simulink model "Regressao6"  (R2012b)
settings: Solver=FixedStepDiscrete  SolverMode=SingleTasking  StartTime=0.0  StopTime=limSim  FixedStep=ts  RelTol=1e-3
libraries: xbsIndex_r4 x51, roblocks x1
settings Model: Creator=snata  LastModifiedBy=snata

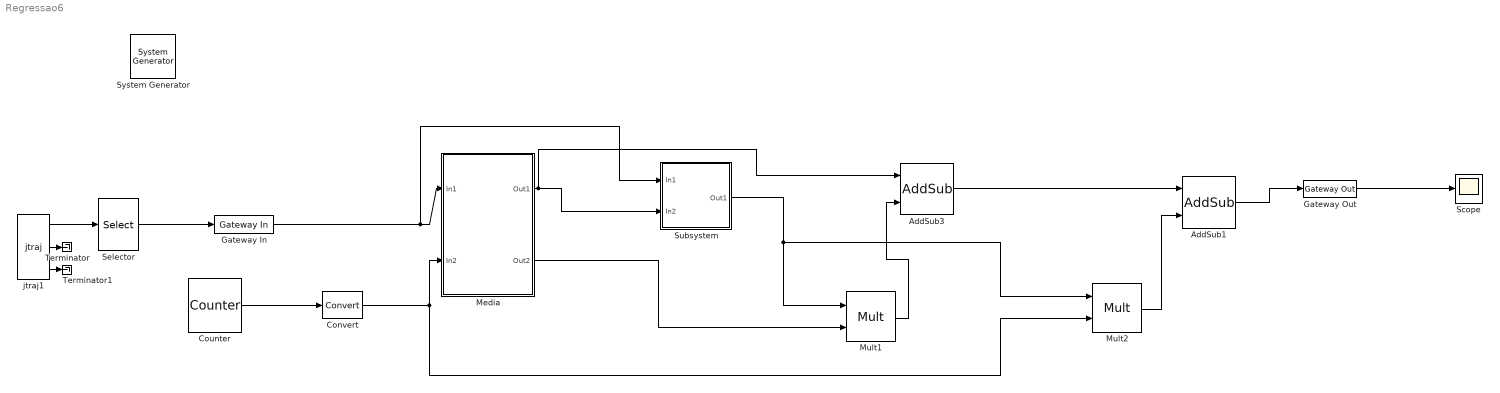
== system Regressao6 ==
  " System Generator" : xbsIndex_r4/ System Generator  Tag=genX  xilinxfamily=virtex6  part=xc6vlx240t  speed=-1  package=ff1156  synthesis_tool=XST  clock_wrapper=Clock Enables  directory=./netlist  proj_type=Project Navigator  Synth_file=XST Defaults  Impl_file=ISE Defaults  testbench=off  simulink_period=ts  sysclk_period=10  dcm_input_clock_period=10  incr_netlist=off  trim_vbits=Everywhere in SubSystem  dbl_ovrd=According to Block Masks  core_generation=According to Block Masks  run_coregen=off  deprecated_control=off  eval_field=0  block_type=sysgen
  AddSub1 : xbsIndex_r4/AddSub  mode=Addition  use_carryin=off  use_carryout=off  en=off  latency=0  precision=Full  arith_type=Unsigned  n_bits=16  bin_pt=14  quantization=Truncate  overflow=Wrap  dbl_ovrd=off  use_behavioral_HDL=off  hw_selection=Fabric  pipelined=off  block_type=addsub
  AddSub3 : xbsIndex_r4/AddSub  mode=Subtraction  use_carryin=off  use_carryout=off  en=off  latency=0  precision=Full  arith_type=Unsigned  n_bits=16  bin_pt=14  quantization=Truncate  overflow=Wrap  dbl_ovrd=off  use_behavioral_HDL=off  hw_selection=Fabric  pipelined=off  block_type=addsub
  Convert : xbsIndex_r4/Convert  gui_display_data_type=Floating-point  arith_type=Floating-point  n_bits=16  bin_pt=14  float_type=Single  exp_bits=8  fraction_bits=24  quantization=Truncate  overflow=Wrap  en=off  latency=0  dbl_ovrd=off  pipeline=off  block_type=convert
  Counter : xbsIndex_r4/Counter  cnt_type=Free Running  cnt_to=Inf  operation=Up  start_count=0  cnt_by_val=1  arith_type="Signed  (2's comp)"  n_bits=32  bin_pt=1  load_pin=off  rst=off  en=off  explicit_period=on  period=ts  dbl_ovrd=off  use_behavioral_HDL=off  implementation=Fabric  block_type=counter
  Gateway In : xbsIndex_r4/Gateway In  gui_display_data_type=Floating-point  arith_type=Floating-point  n_bits=16  bin_pt=14  preci_type=Single  exp_width=8  frac_width=24  quantization="Round  (unbiased: +/- Inf)"  overflow=Saturate  period=ts  dbl_ovrd=off  timing_constraint=None  locs_specified=off  LOCs={}  UseAsADC=off  ADCChannel='1'  inherit_from_input=off  hdl_port=on  block_type=gatewayin
  Gateway Out : xbsIndex_r4/Gateway Out  inherit_from_input=off  hdl_port=on  timing_constraint=None  locs_specified=off  LOCs={}  UseAsDAC=off  DACChannel='1'  block_type=gatewayout
  "Media " : Subsystem
  Mult1 : xbsIndex_r4/Mult  precision=Full  arith_type="Signed  (2's comp)"  n_bits=16  bin_pt=14  quantization=Truncate  overflow=Wrap  en=off  latency=0  dbl_ovrd=off  use_behavioral_HDL=off  opt=Speed  use_embedded=on  optimum_pipeline=off  pipeline=on  use_rpm=on  placement_style=Triangular  block_type=mult
  Mult2 : xbsIndex_r4/Mult  precision=Full  arith_type="Signed  (2's comp)"  n_bits=16  bin_pt=14  quantization=Truncate  overflow=Wrap  en=off  latency=0  dbl_ovrd=off  use_behavioral_HDL=off  opt=Speed  use_embedded=on  optimum_pipeline=off  pipeline=on  use_rpm=on  placement_style=Triangular  block_type=mult
  Scope : Scope
      settings: YMin=5.55112e-17  YMax=1.6
  Selector : Selector  InputPortWidth=3  IndexOptions=Index vector (dialog)  Indices=[1]  OutputSizes=1
  Subsystem : Subsystem
  Terminator : Terminator
  Terminator1 : Terminator
  jtraj1 : roblocks/Trajectory/jtraj  q0=[0 -pi/2 pi]  qf=[pi/2 pi/4 pi/2]  tmax=limSim  ts=ts
  wires:
  Selector/1 -> Gateway In/1
  jtraj1/1 -> Selector/1
  Gateway In/1 -> Subsystem/1(In1), "Media "/1(In1)
  AddSub1/1 -> Gateway Out/1
  Gateway Out/1 -> Scope/1
  "Media "/1(Out1) -> AddSub3/1, Subsystem/2(In2)
  Counter/1 -> Convert/1
  Convert/1 -> "Media "/2(In2), Mult2/2
  Mult1/1 -> AddSub3/2
  AddSub3/1 -> AddSub1/1
  Mult2/1 -> AddSub1/2
  Subsystem/1(Out1) -> Mult2/1, Mult1/1
  "Media "/2(Out2) -> Mult1/2
  jtraj1/2 -> Terminator/1
  jtraj1/3 -> Terminator1/1

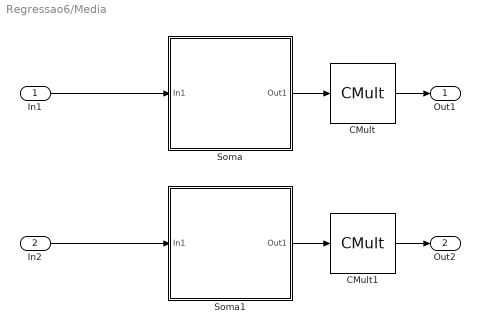
== system Regressao6/Media  ==
  In1 : Inport
  In2 : Inport  Port=2
  CMult : xbsIndex_r4/CMult  const=1/7  gui_display_data_type=Floating-point  const_n_bits=16  const_bin_pt=14  float_type=Single  exp_bits=8  fraction_bits=24  en=off  latency=0  precision=Full  arith_type="Signed  (2's comp)"  n_bits=16  bin_pt=14  quantization=Truncate  overflow=Wrap  dbl_ovrd=off  use_behavioral_HDL=off  mem_type=Distributed RAM  pipeline=off  block_type=cmult
  CMult1 : xbsIndex_r4/CMult  const=1/7  gui_display_data_type=Floating-point  const_n_bits=16  const_bin_pt=14  float_type=Single  exp_bits=8  fraction_bits=24  en=off  latency=0  precision=Full  arith_type="Signed  (2's comp)"  n_bits=16  bin_pt=14  quantization=Truncate  overflow=Wrap  dbl_ovrd=off  use_behavioral_HDL=off  mem_type=Distributed RAM  pipeline=off  block_type=cmult
  Soma : Subsystem
  Soma1 : Subsystem
  Out1 : Outport
  Out2 : Outport  Port=2
  wires:
  In1/1 -> Soma/1(In1)
  Soma/1(Out1) -> CMult/1
  CMult/1 -> Out1/1
  In2/1 -> Soma1/1(In1)
  Soma1/1(Out1) -> CMult1/1
  CMult1/1 -> Out2/1

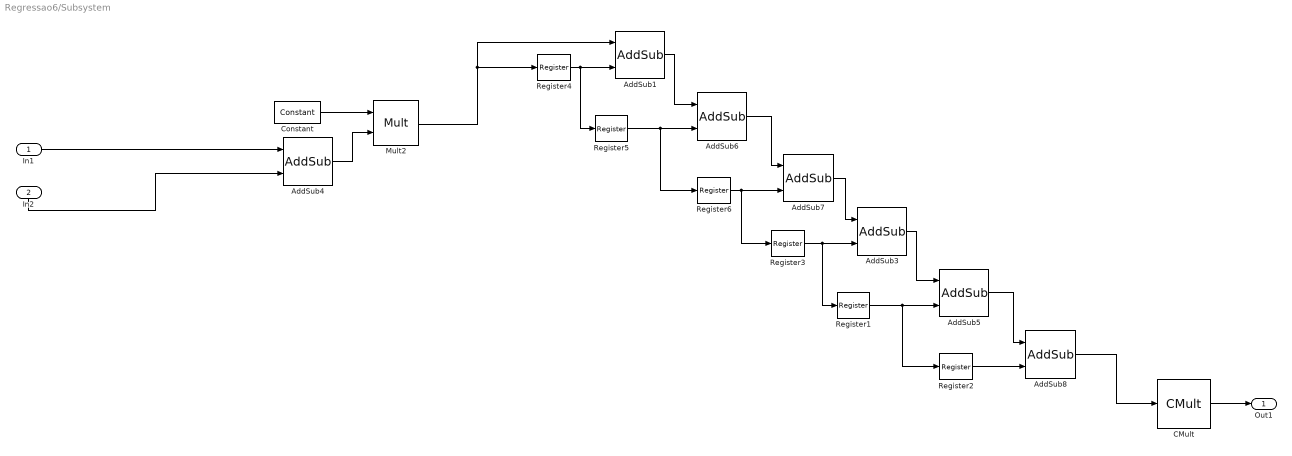
== system Regressao6/Subsystem ==
  In1 : Inport
  In2 : Inport  Port=2
  AddSub{1,3,5..8} (6 alike) : xbsIndex_r4/AddSub  mode=Addition  use_carryin=off  use_carryout=off  en=off  latency=0  precision=Full  arith_type=Unsigned  n_bits=16  bin_pt=14  quantization=Truncate  overflow=Wrap  dbl_ovrd=off  use_behavioral_HDL=off  hw_selection=Fabric  pipelined=off  block_type=addsub
  AddSub4 : xbsIndex_r4/AddSub  mode=Subtraction  use_carryin=off  use_carryout=off  en=off  latency=0  precision=Full  arith_type=Unsigned  n_bits=16  bin_pt=14  quantization=Truncate  overflow=Wrap  dbl_ovrd=off  use_behavioral_HDL=off  hw_selection=Fabric  pipelined=off  block_type=addsub
  CMult : xbsIndex_r4/CMult  const=1/9  gui_display_data_type=Floating-point  const_n_bits=16  const_bin_pt=14  float_type=Single  exp_bits=8  fraction_bits=24  en=off  latency=0  precision=Full  arith_type="Signed  (2's comp)"  n_bits=16  bin_pt=14  quantization=Truncate  overflow=Wrap  dbl_ovrd=off  use_behavioral_HDL=off  mem_type=Distributed RAM  pipeline=off  block_type=cmult
  Constant : xbsIndex_r4/Constant  const=3  gui_display_data_type=Floating-point  arith_type=Floating-point  n_bits=16  bin_pt=14  preci_type=Single  exp_width=8  frac_width=24  explicit_period=off  period=1  equ=P=C  opselect=C  inp2=PCIN>>17  opr=+  inp1=P  carry=CIN  dbl_ovrd=off  block_type=constant
  Mult2 : xbsIndex_r4/Mult  precision=Full  arith_type="Signed  (2's comp)"  n_bits=16  bin_pt=14  quantization=Truncate  overflow=Wrap  en=off  latency=0  dbl_ovrd=off  use_behavioral_HDL=off  opt=Speed  use_embedded=on  optimum_pipeline=off  pipeline=on  use_rpm=on  placement_style=Triangular  block_type=mult
  Register{1..6} (6 alike) : xbsIndex_r4/Register  init=0  rst=off  en=off  dbl_ovrd=off  block_type=register
  Out1 : Outport
  wires:
  CMult/1 -> Out1/1
  AddSub4/1 -> Mult2/2
  In1/1 -> AddSub4/1
  In2/1 -> AddSub4/2
  AddSub8/1 -> CMult/1
  Mult2/1 -> AddSub1/1, Register4/1
  AddSub6/1 -> AddSub7/1
  AddSub1/1 -> AddSub6/1
  Register4/1 -> Register5/1, AddSub1/2
  Register5/1 -> Register6/1, AddSub6/2
  Register6/1 -> Register3/1, AddSub7/2
  AddSub5/1 -> AddSub8/1
  AddSub3/1 -> AddSub5/1
  Register3/1 -> Register1/1, AddSub3/2
  Register1/1 -> Register2/1, AddSub5/2
  Register2/1 -> AddSub8/2
  AddSub7/1 -> AddSub3/1
  Constant/1 -> Mult2/1

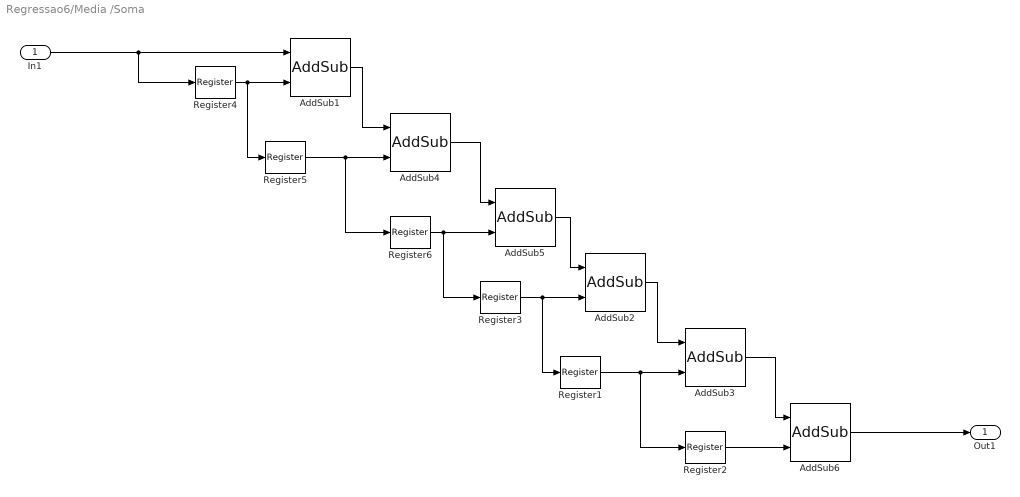
== system Regressao6/Media /Soma ==
  In1 : Inport
  AddSub{1..6} (6 alike) : xbsIndex_r4/AddSub  mode=Addition  use_carryin=off  use_carryout=off  en=off  latency=0  precision=Full  arith_type=Unsigned  n_bits=16  bin_pt=14  quantization=Truncate  overflow=Wrap  dbl_ovrd=off  use_behavioral_HDL=off  hw_selection=Fabric  pipelined=off  block_type=addsub
  Register{1..6} (6 alike) : xbsIndex_r4/Register  init=0  rst=off  en=off  dbl_ovrd=off  block_type=register
  Out1 : Outport
  wires:
  In1/1 -> Register4/1, AddSub1/1
  AddSub4/1 -> AddSub5/1
  AddSub1/1 -> AddSub4/1
  Register4/1 -> Register5/1, AddSub1/2
  Register5/1 -> Register6/1, AddSub4/2
  Register6/1 -> Register3/1, AddSub5/2
  AddSub3/1 -> AddSub6/1
  AddSub2/1 -> AddSub3/1
  Register3/1 -> Register1/1, AddSub2/2
  Register1/1 -> Register2/1, AddSub3/2
  Register2/1 -> AddSub6/2
  AddSub5/1 -> AddSub2/1
  AddSub6/1 -> Out1/1

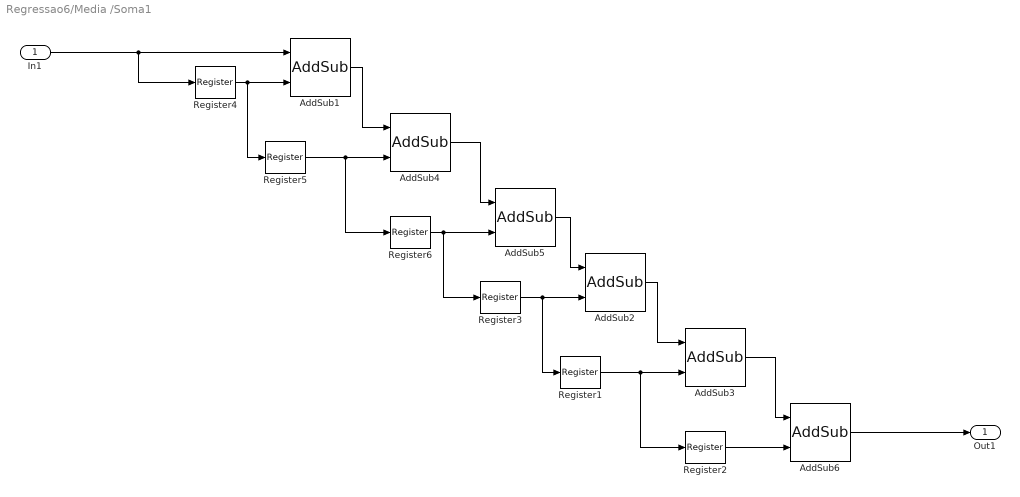
== system Regressao6/Media /Soma1 ==
  In1 : Inport
  AddSub{1..6} (6 alike) : xbsIndex_r4/AddSub  mode=Addition  use_carryin=off  use_carryout=off  en=off  latency=0  precision=Full  arith_type=Unsigned  n_bits=16  bin_pt=14  quantization=Truncate  overflow=Wrap  dbl_ovrd=off  use_behavioral_HDL=off  hw_selection=Fabric  pipelined=off  block_type=addsub
  Register{1..6} (6 alike) : xbsIndex_r4/Register  init=0  rst=off  en=off  dbl_ovrd=off  block_type=register
  Out1 : Outport
  wires:
  AddSub6/1 -> Out1/1
  AddSub5/1 -> AddSub2/1
  Register2/1 -> AddSub6/2
  Register1/1 -> AddSub3/2, Register2/1
  Register3/1 -> AddSub2/2, Register1/1
  AddSub2/1 -> AddSub3/1
  AddSub3/1 -> AddSub6/1
  Register6/1 -> AddSub5/2, Register3/1
  Register5/1 -> AddSub4/2, Register6/1
  Register4/1 -> AddSub1/2, Register5/1
  AddSub1/1 -> AddSub4/1
  AddSub4/1 -> AddSub5/1
  In1/1 -> AddSub1/1, Register4/1
